simulink model "shell_eco_mainV2"  (R2023b)
settings: Solver=VariableStepAuto  StartTime=0.0  StopTime=60  RelTol=1e-3
undefined symbols (not defined in the file): A, Cd, Crr, effic_drive, g, G, LHV, m, r_w, rho, RPM_idle, RPM_max, v0, x0
settings Model: Creator=canfi  LastModifiedBy=canfi

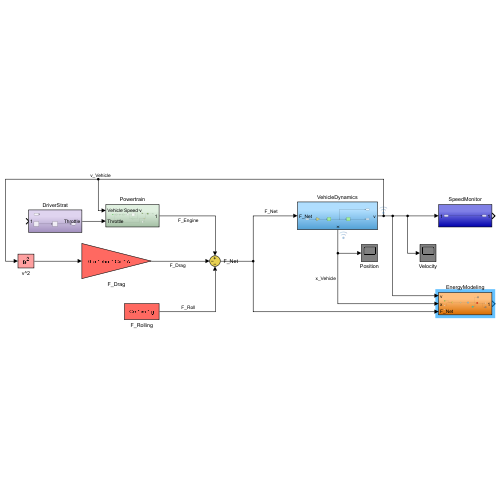
[thumbnail: Simulink's stored preview of the top-level diagram]
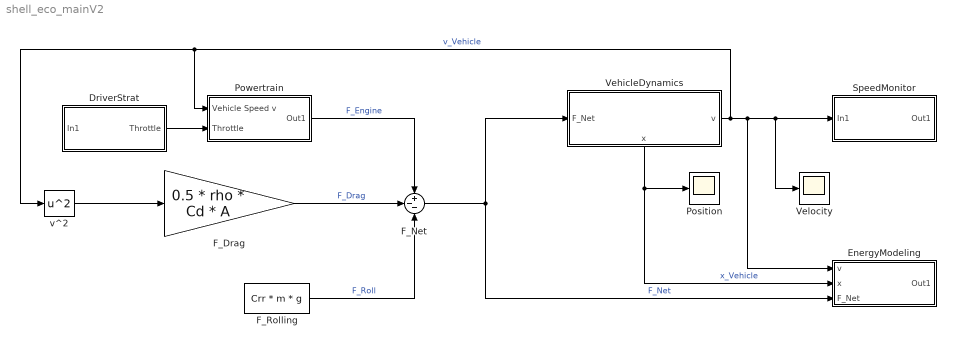
== system shell_eco_mainV2 ==
  DriverStrat : Subsystem
  EnergyModeling : Subsystem
  F_Drag : Gain  Gain=0.5 * rho * Cd * A
  F_Net : Sum  Inputs=+--
  F_Rolling : Constant  Value=Crr * m * g
  Position : Scope
  Powertrain : Subsystem
  SpeedMonitor : Subsystem
  VehicleDynamics : Subsystem
      settings: PortSchema="{\"entries\":[{\"content\":{\"sides\":[{\"content\":{\"connectorIds\":[\"In1\"]},\"type\":\"ConnectorPlacement.EquallySpacedRectSide\",\"uuid\":\"dfdfb956-2909-41e2-ad74-eec43401073f\"},{\"content\":{\"connectorIds\":[\"Out1\"],\"side\":\"RIGHT\"},\"type\":\"ConnectorPlacement.EquallySpacedRectSide\",\"uuid\":\"11842bdc-6931-40ed-a403-b6947f0a89a0\"},{\"content\":{\"side\":\"TOP\"},\"type\":\"ConnectorPlacement.EquallySpacedRectSide\",\"uuid\":\"79a25e54-4e3e-453f-b478-21948a5fad51\"},{\"content\":{\"connectorIds\":[\"Out2\"],\"side\":\"BOTTOM\"},\"type\":\"ConnectorPlacement.EquallySpacedRectSide\",\"uuid\":\"b1ef2620-ee40-4a96-8fe4-d7ac3411631d\"}]},\"type\":\"ConnectorPlacement.EquallySpacedConnector\",\"uuid\":\"a04151ff-9342-40bb-a5c2-12dc5cb0586b\"}],\"packageUris\":[\"http://schema.mathworks.com/mf0/Connector/R2020b\"],\"version\":\"1.0\"}"
  Velocity : Scope
  v^2 : Math  Operator=square
  wires:
  DriverStrat/1(Throttle) -> Powertrain/2(Throttle)
  VehicleDynamics/2(x) -> EnergyModeling/2(x), Position/1  "x_Vehicle"
  VehicleDynamics/1(v) -> SpeedMonitor/1(In1), Velocity/1, EnergyModeling/1(v), Powertrain/1(Vehicle Speed v), v^2/1  "v_Vehicle"
  Powertrain/1(Out1) -> F_Net/1  "F_Engine"
  v^2/1 -> F_Drag/1
  F_Net/1 -> EnergyModeling/3(F_Net), VehicleDynamics/1(F_Net)  "F_Net"
  F_Rolling/1 -> F_Net/3  "F_Roll"
  F_Drag/1 -> F_Net/2  "F_Drag"

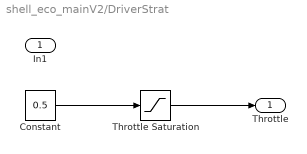
== system shell_eco_mainV2/DriverStrat ==
  In1 : Inport
  Constant : Constant  Value=0.5
  Throttle Saturation : Saturate  UpperLimit=1  LowerLimit=0
  Throttle : Outport
  wires:
  Constant/1 -> Throttle Saturation/1
  Throttle Saturation/1 -> Throttle/1

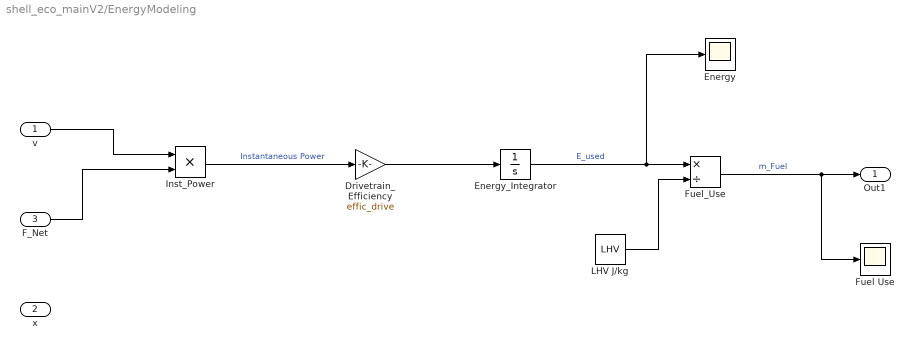
== system shell_eco_mainV2/EnergyModeling ==
  v : Inport
  x : Inport  Port=2
  F_Net : Inport  Port=3
  Drivetrain_Efficiency : Gain  Gain=effic_drive
  Energy : Scope
  Energy_Integrator : Integrator
  Fuel Use : Scope
  Fuel_Use : Product  Inputs=*/
  Inst_Power : Product
  LHV J/kg : Constant  Value=LHV
  Out1 : Outport
  wires:
  v/1 -> Inst_Power/1
  F_Net/1 -> Inst_Power/2
  Inst_Power/1 -> Drivetrain_Efficiency/1  "Instantaneous Power"
  Energy_Integrator/1 -> Fuel_Use/1, Energy/1  "E_used"
  Drivetrain_Efficiency/1 -> Energy_Integrator/1
  LHV J/kg/1 -> Fuel_Use/2
  Fuel_Use/1 -> Out1/1, Fuel Use/1  "m_Fuel"

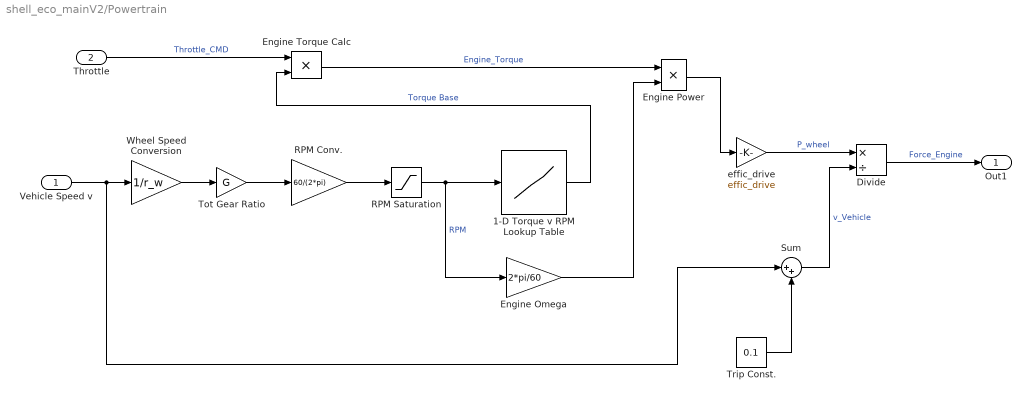
== system shell_eco_mainV2/Powertrain ==
  Vehicle Speed v : Inport
  Throttle : Inport  Port=2
  1-D Torque v RPM Lookup Table : Lookup_n-D  NumberOfTableDimensions=1  BreakpointsForDimension1=[2000 4000 6000 8000]  Table=[2.1 2.8 3.2 2.7]  ExtrapMethod=Clip  InternalRulePriority=Speed  RndMeth=Simplest
  Divide : Product  Inputs=*/
  Engine Omega : Gain  Gain=2*pi/60
  Engine Power : Product
  Engine Torque Calc : Product
  RPM Conv. : Gain  Gain=60/(2*pi)
  RPM Saturation : Saturate  UpperLimit=RPM_max  LowerLimit=RPM_idle
  Sum : Sum  Inputs=|++
  Tot Gear Ratio : Gain  Gain=G
  Trip Const. : Constant  Value=0.1
  Wheel Speed Conversion : Gain  Gain=1/r_w
  effic_drive : Gain  Gain=effic_drive
  Out1 : Outport
  wires:
  Wheel Speed Conversion/1 -> Tot Gear Ratio/1
  Tot Gear Ratio/1 -> RPM Conv./1
  Vehicle Speed v/1 -> Wheel Speed Conversion/1, Sum/1
  RPM Conv./1 -> RPM Saturation/1
  1-D Torque v RPM Lookup Table/1 -> Engine Torque Calc/2  "Torque Base"
  Throttle/1 -> Engine Torque Calc/1  "Throttle_CMD"
  Engine Torque Calc/1 -> Engine Power/1  "Engine_Torque"
  Engine Omega/1 -> Engine Power/2
  Engine Power/1 -> effic_drive/1
  effic_drive/1 -> Divide/1  "P_wheel"
  Trip Const./1 -> Sum/2
  Sum/1 -> Divide/2  "v_Vehicle"
  Divide/1 -> Out1/1  "Force_Engine"
  RPM Saturation/1 -> Engine Omega/1, 1-D Torque v RPM Lookup Table/1  "RPM"

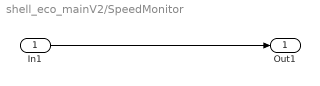
== system shell_eco_mainV2/SpeedMonitor ==
  In1 : Inport
  Out1 : Outport
  wires:
  In1/1 -> Out1/1

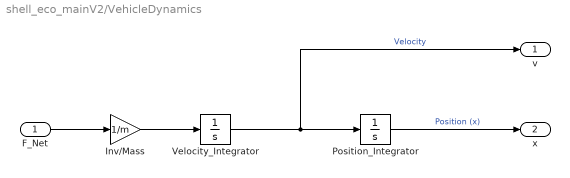
== system shell_eco_mainV2/VehicleDynamics ==
  F_Net : Inport
  Inv/Mass : Gain  Gain=1/m
  Position_Integrator : Integrator  InitialCondition=x0
  Velocity_Integrator : Integrator  InitialCondition=v0
  v : Outport
  x : Outport  Port=2
  wires:
  Inv/Mass/1 -> Velocity_Integrator/1
  Velocity_Integrator/1 -> v/1, Position_Integrator/1  "Velocity"
  Position_Integrator/1 -> x/1  "Position (x)"
  F_Net/1 -> Inv/Mass/1
